simulink model "stateflow_example"  (R2020a)
settings: Solver=VariableStepAuto  StartTime=0.0  StopTime=10.0  RelTol=1e-3
libraries: robotlib x1
settings Model: Creator=ivory  LastModifiedBy=ivory

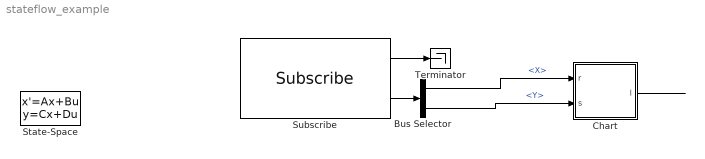
== system stateflow_example ==
  Bus Selector : BusSelector  OutputSignals=X,Y
  Chart : Stateflow chart  TreatAsAtomicUnit=on
  State-Space : StateSpace  InitialCondition=0
  Subscribe : robotlib/Subscribe  topicSource=Select from ROS network  topic=/my_topic  messageType=geometry_msgs/Point  sampleTime=-1  messageQueueLength=1
  Terminator : Terminator
  wires:
  Subscribe/1 -> Terminator/1
  Subscribe/2 -> Bus Selector/1
  Bus Selector/1 -> Chart/1(r)  "<X>"
  Bus Selector/2 -> Chart/2(s)  "<Y>"
  Chart/1(l) -> ?

== stateflow chart stateflow_example/Chart ==
  state State_1
    entry: m = callme(r, s); i = 0;
    during: s = r(i) + s;l = s + 1;
    exit: s = r - s;
  state State_2
  (default) -> State_1
  State_1 -> State_2 [order 2] : [r == s && s >= 1]
  State_1 -> State_2 [order 1] : [s > 10]{r = 0}
  State_2 -> State_1
  data: r function_input; s function_input; ret function_output; p local; q local; r input size=5; s input double; l output; m local
  function ret = callme(r, s):
    | function ret = callme(r, s)
    | 
    | ret = r*s;
